simulink model "EV_project"  (R2024a)
settings: Solver=FixedStepAuto  StartTime=0.0  StopTime=250  FixedStep=5e-6  RelTol=1e-6  AbsTol=1e-6
model workspace (MATLAB code in the model file):
  | Rw = 0.2736; % radius of vehicle(m)
  | GVM = 225; % gross vehicle mass(kg)
  | GVW = GVM*9.8; % gross vehicle weight(kg.m/s^2)
  | Crf = 0.012; % coeff of rolling resistance
  | slope_angle = 0; % slope angle in radian
  | Af = 1.73; % frontal Area(m^2)
  | Cd = 0.4; % coeff of drag
  | gear_ratio = 6;
  | trans_eff = 0.95;
  | motor_eff = 0.93;
  | mc_eff = 0.95;
  | Bv = 300; % Battery Voltage(V)
  | Cv = 3.6; % Cell voltage(V)
  | Cc = 31; % Cell capacity(Ah)
  | lap_distance = 0.787; % distance of one lap(km)
  | range = 20; % range of vehicle in single charge
  | time = 60; % time required to complete one lap
  | air_density = 1.225;
libraries: spsDCVoltageSourceLib x1, spsGroundLib x1, slpidlib x1, spsPermanentMagnetSynchronousMachineLib x1, spsThreePhaseVIMeasurementLib x1, spsUniversalBridgeLib x1, simulink x1, spspowerguiLib x1
settings Model: SimulationMode=accelerator  Creator=mohda  LastModifiedBy=MD. ADEEN ASHRAF
settings SolverCC: AlgebraicLoopSolver=TrustRegion
settings RTWCC: GPUComputeCapability=3.5

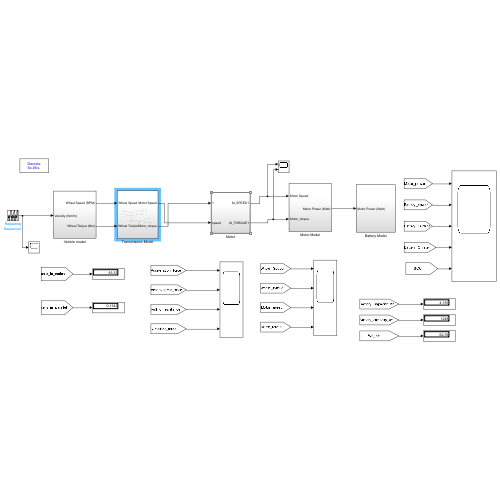
[thumbnail: Simulink's stored preview of the top-level diagram]
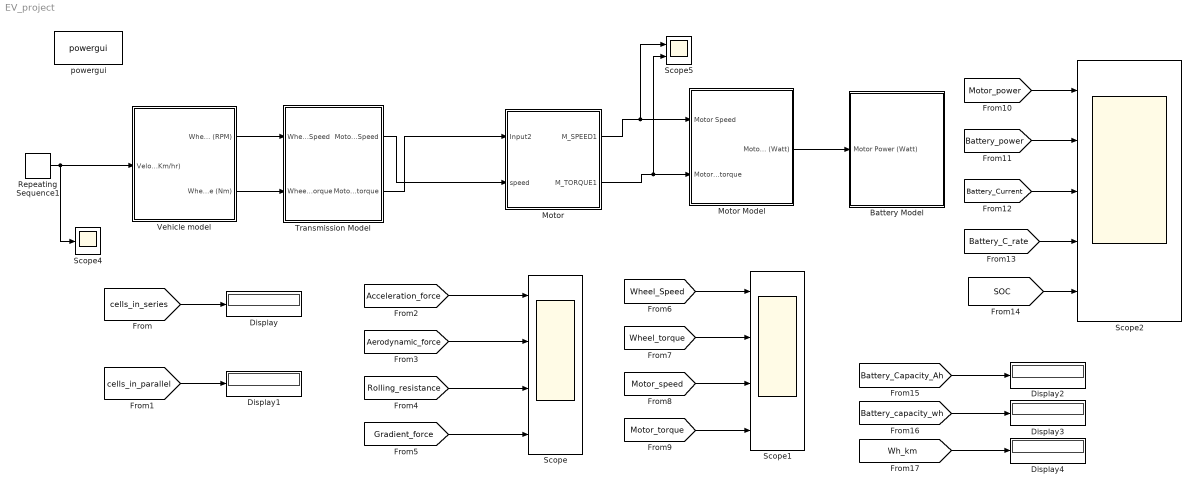
== system EV_project ==
  Battery Model : Subsystem
  Display{,1..4} (5 alike) : Display
  Motor : Subsystem
  Motor Model : Subsystem
  Repeating Sequence1 : simulink/Sources/Repeating Sequence  rep_seq_t=|  rep_seq_y=|
      rep_seq_t=|
      | [0
      | 1
      | 2
      | 3
      | 4
      | 5
      | 6
      | 7
      | 8
      | 9
      | 10
      | 11
      | 12
      | 13
      | 14
      | 15
      | 16
      | 17
      | 18
      | 19
      | 20
      | 21
      | 22
      | 23
      | 24
      | 25
      | 26
      | 27
      | 28
      | 29
      | 30
      | 31
      | 32
      | 33
      | 34
      | 35
      | 36
      | 37
      | 38
      | 39
      | 40
      | 41
      | 42
      | 43
      | 44
      | 45
      | 46
      | 47
      | 48
      | 49
      | 50
      | 51
      | 52
      | 53
      | 54
      | 55
      | 56
      | 57
      | 58
      | 59
      | 60
      | 61
      | 62
      | 63
      | 64
      | 65
      | 66
      | 67
      | 68
      | 69
      | 70
      | 71
      | 72
      | 73
      | 74
      | 75
      | 76
      | 77
      | 78
      | 79
      | 80
      | 81
      | 82
      | 83
      | 84
      | 85
      | 86
      | 87
      | 88
      | 89
      | 90
      | 91
      | 92
      | 93
      | 94
      | 95
      | 96
      | 97
      | 98
      | 99
      | 100
      | 101
      | 102
      | 103
      | 104
      | 105
      | 106
      | 107
      | 108
      | 109
      | 110
      | 111
      | 112
      | 113
      | 114
      | 115
      | 116
      | 117
      | 118
      | 119
      | 120
      | 121
      | 122
      | 123
      | 124
      | 125
      | 126
      | 127
      | 128
      | 129
      | 130
      | 131
      | 132
      | 133
      | 134
      | 135
      | 136
      | 137
      | 138
      | 139
      | 140
      | 141
      | 142
      | 143
      | 144
      | 145
      | 146
      | 147
      | 148
      | 149
      | 150
      | 151
      | 152
      | 153
      | 154
      | 155
      | 156
      | 157
      | 158
      | 159
      | 160
      | 161
      | 162
      | 163
      | 164
      | 165
      | 166
      | 167
      | 168
      | 169
      | 170
      | 171
      | 172
      | 173
      | 174
      | 175
      | 176
      | 177
      | 178
      | 179
      | 180
      | 181
      | 182
      | 183
      | 184
      | 185
      | 186
      | 187
      | 188
      | 189
      | 190
      | 191
      | 192
      | 193
      | 194
      | 195
      | 196
      | 197
      | 198
      | 199
      | 200
      | 201
      | 202
      | 203
      | 204
      | 205
      | 206
      | 207
      | 208
      | 209
      | 210
      | 211
      | 212
      | 213
      | 214
      | 215
      | 216
      | 217
      | 218
      | 219
      | 220
      | 221
      | 222
      | 223
      | 224
      | 225
      | 226
      | 227
      | 228
      | 229
      | 230
      | 231
      | 232
      | 233
      | 234
      | 235
      | 236
      | 237
      | 238
      | 239
      | 240
      | 241
      | 242
      | 243
      | 244
      | 245
      | 246
      | 247
      | 248
      | 249
      | 250 ]
      rep_seq_y=|
      | [0
      | 0
      | 0
      | 0
      | 0
      | 0
      | 0
      | 0
      | 0
      | 0
      | 0
      | 0
      | 3
      | 5.9
      | 8.6
      | 11.5
      | 14.3
      | 16.9
      | 17.3
      | 18.1
      | 20.7
      | 21.7
      | 22.4
      | 22.5
      | 22.1
      | 21.5
      | 20.9
      | 20.4
      | 19.8
      | 17
      | 14.9
      | 14.9
      | 15.2
      | 15.5
      | 16
      | 17.1
      | 19.1
      | 21.1
      | 22.7
      | 22.9
      | 22.7
      | 22.6
      | 21.3
      | 19
      | 17.1
      | 15.8
      | 15.8
      | 17.7
      | 19.8
      | 21.6
      | 23.2
      | 24.2
      | 24.6
      | 24.9
      | 25
      | 25.7
      | 26.1
      | 26.7
      | 27.5
      | 28.6
      | 29.3
      | 29.8
      | 30.1
      | 30.4
      | 30.7
      | 30.7
      | 30.5
      | 30.4
      | 30.3
      | 30.4
      | 30.8
      | 30.4
      | 29.9
      | 29.5
      | 29.8
      | 30.3
      | 30.7
      | 30.9
      | 31
      | 30.9
      | 30.4
      | 29.8
      | 29.9
      | 30.2
      | 30.7
      | 31.2
      | 31.8
      | 32.2
      | 32.4
      | 32.2
      | 31.7
      | 28.6
      | 25.1
      | 21.6
      | 18.1
      | 14.6
      | 11.1
      | 7.6
      | 4.1
      | 0.6
      | 0
      | 0
      | 0
      | 0
      | 0
      | 3.3
      | 6.6
      | 9.9
      | 13.2
      | 16.5
      | 19.8
      | 22.2
      | 24.3
      | 25.8
      | 26.4
      | 25.7
      | 25.1
      | 24.7
      | 25.2
      | 25.4
      | 27.2
      | 26.5
      | 24
      | 22.7
      | 19.4
      | 17.7
      | 17.2
      | 18.1
      | 18.6
      | 20
      | 20.7
      | 21.7
      | 22.4
      | 22.5
      | 22.1
      | 21.5
      | 20.9
      | 20.4
      | 19.8
      | 17
      | 17.1
      | 15.8
      | 15.8
      | 17.7
      | 19.8
      | 21.6
      | 22.2
      | 24.5
      | 24.7
      | 24.8
      | 24.7
      | 24.6
      | 24.6
      | 25.1
      | 25.6
      | 25.7
      | 25.4
      | 24.9
      | 25
      | 25.4
      | 26
      | 26
      | 25.7
      | 26.1
      | 26.7
      | 27.3
      | 30.5
      | 33.5
      | 36.2
      | 37.3
      | 39.3
      | 40.5
      | 42.1
      | 43.5
      | 45.1
      | 46
      | 46.8
      | 47.5
      | 47.5
      | 47.3
      | 47.2
      | 47.2
      | 47.4
      | 47.9
      | 48.5
      | 49.1
      | 49.5
      | 50
      | 50.6
      | 51
      | 51.5
      | 52.2
      | 53.2
      | 54.1
      | 54.6
      | 54.9
      | 55
      | 54.9
      | 54.6
      | 54.6
      | 54.8
      | 55.1
      | 55.5
      | 55.7
      | 56.1
      | 56.3
      | 56.6
      | 56.7
      | 56.7
      | 56.3
      | 56
      | 55
      | 53.4
      | 51.6
      | 51.8
      | 52.1
      | 52.5
      | 53
      | 53.5
      | 54
      | 54.9
      | 55.4
      | 55.6
      | 56
      | 56
      | 55.8
      | 55.2
      | 54.5
      | 53.6
      | 52.5
      | 51.5
      | 50.5
      | 48
      | 44.5
      | 41
      | 37.5
      | 34
      | 30.5
      | 27
      | 23.5
      | 20
      | 16.5
      | 13
      | 9.5
      | 6
      | 2.5
      | 0
      | 0
      | 0
      | 0
      | 0 ]
  Scope : Scope  NumInputPorts=4
  Scope1 : Scope  NumInputPorts=4
  Scope2 : Scope  NumInputPorts=5
  Scope4 : Scope
  Scope5 : Scope  NumInputPorts=2
  Transmission Model : Subsystem
  Vehicle model : Subsystem
  powergui : spspowerguiLib/powergui  Priority=1  SimulationMode=Discrete  SampleTime=5e-6  frequency=60  Iterations=50  frequencyindice=0  Pbase=100e6  ErrMax=1e-4  UnitsV=kV  UnitsW=MW  buscounter=0  FunctionMessages=off  echomessages=off  EnableUseOfTLC=off  CurrentSourceSwitches=off  DisableSnubberDevices=off  DisableRonSwitches=off  DisableVfSwitches=off  DisplayEquations=off  AutomaticDiscreteSolvers=off  SolverType=Tustin/Backward Euler (TBE)  Interpol=off  ExternalGateDelay=off  methode=off  Ts=100  x0status=blocks  SPID=on  SwTol=0  HookPort=off  NonlinearTolerance=1e-4  nMaxIteration=100  ContinueOnMaxIteration=off  RestoreLinks=warning  ResistiveCurrentMeasurement=off  Frange=[0:2:500]  Ylog=off  Xlog=on  ShowGrid=off  save=off  variable=ZData  structure=0  ZoomFFT=off  StartTime=0.0  cycles=1  DisplayStyle=1  fundamental=60  FreqAxis=off  MaxFrequency=1000  frequencyindicesteady=1  RmsSteady=1  display=off
  wires:
  Motor Model/1(Motor Power (Watt)) -> Battery Model/1(Motor Power (Watt))
  [cells_in_series] -> Display/1
  [cells_in_parallel] -> Display1/1
  [Acceleration_force] -> Scope/1
  [Aerodynamic_force] -> Scope/2
  [Rolling_resistance] -> Scope/3
  [Gradient_force] -> Scope/4
  [Wheel_Speed] -> Scope1/1
  [Wheel_torque] -> Scope1/2
  [Motor_speed] -> Scope1/3
  [Motor_torque] -> Scope1/4
  [Battery_C_rate] -> Scope2/4
  [SOC] -> Scope2/5
  [Battery_Current] -> Scope2/3
  [Battery_power] -> Scope2/2
  [Motor_power] -> Scope2/1
  [Battery_Capacity_Ah] -> Display2/1
  [Battery_capacity_wh] -> Display3/1
  [Wh_km] -> Display4/1
  Vehicle model/1(Wheel Speed (RPM)) -> Transmission Model/1(Wheel Speed)
  Vehicle model/2(Wheel Torque (Nm)) -> Transmission Model/2(Wheel Torque)
  Motor/1(M_SPEED1) -> Scope5/1, Motor Model/1(Motor Speed)
  Motor/2(M_TORQUE1) -> Scope5/2, Motor Model/2(Motor_torque)
  Transmission Model/1(Motor Speed) -> Motor/2(speed)
  Transmission Model/2(Motor_torque) -> Motor/1(Input2)
  Repeating Sequence1/1 -> Scope4/1, Vehicle model/1(Velocity (Km/hr))

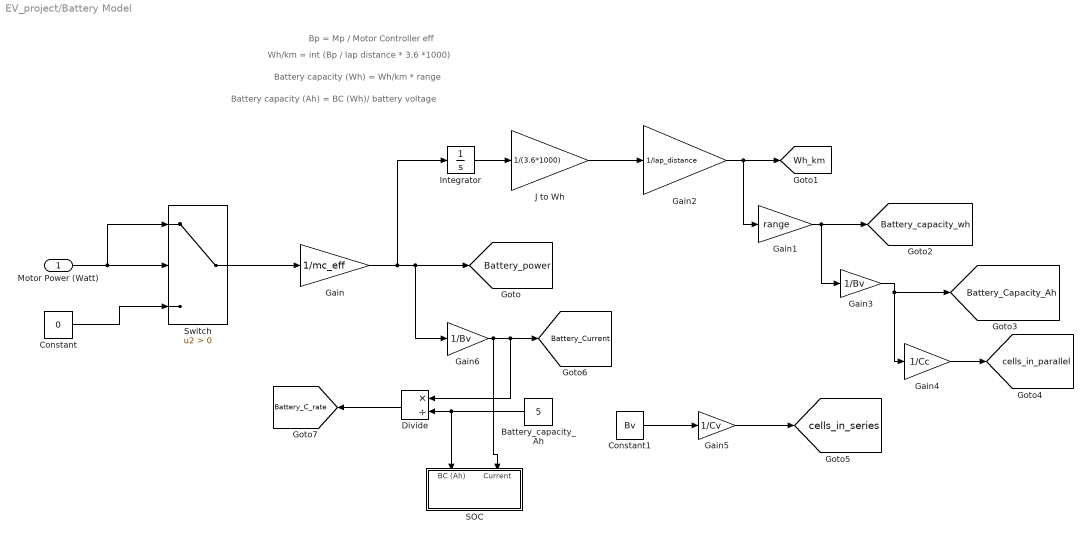
== system EV_project/Battery Model ==
  note: Battery capacity (Ah) = BC (Wh)/ battery voltage
  note: Battery capacity (Wh) = Wh/km * range
  note: Wh/km = int (Bp / lap distance * 3.6 *1000)
  note: Bp = Mp / Motor Controller eff
  Motor Power (Watt) : Inport
  Battery_capacity_Ah : Constant  Value=5
  Constant : Constant  Value=0
  Constant1 : Constant  Value=Bv
  Divide : Product  Inputs=*/
  Gain : Gain  Gain=1/mc_eff
  Gain1 : Gain  Gain=range
  Gain2 : Gain  Gain=1/lap_distance
  Gain3 : Gain  Gain=1/Bv
  Gain4 : Gain  Gain=1/Cc
  Gain5 : Gain  Gain=1/Cv
  Gain6 : Gain  Gain=1/Bv
  Integrator : Integrator
  J to Wh : Gain  Gain=1/(3.6*1000)
  SOC : Subsystem
      settings: PortSchema="{\"entries\":[{\"content\":{\"sides\":[{\"content\":{},\"type\":\"ConnectorPlacement.EquallySpacedRectSide\",\"uuid\":\"2be810da-99f1-4413-b487-e4f7f3ce3b1c\"},{\"content\":{\"side\":\"RIGHT\"},\"type\":\"ConnectorPlacement.EquallySpacedRectSide\",\"uuid\":\"b4550658-4fc6-45c9-b867-461547c61649\"},{\"content\":{\"connectorIds\":[\"In1\",\"In2\"],\"side\":\"TOP\"},\"type\":\"ConnectorPlacement.EquallySpacedRectSide\",\"uuid\":\"a236ffb8-5612-4e8c-b6e9-c7cf7a884809\"}]},\"type\":\"ConnectorPlacement.EquallySpacedConnector\",\"uuid\":\"ea2521ad-76b8-4493-917a-b6fbbcdb85df\"}],\"packageUris\":[\"http://schema.mathworks.com/mf0/Connector/R2020b\"],\"version\":\"1.0\"}"
  Switch : Switch  Criteria=u2 > Threshold  SaturateOnIntegerOverflow=off  InputSameDT=off
  tag scope: Battery_C_rate=global, Battery_Capacity_Ah=global, Battery_Current=global, Battery_capacity_wh=global, Battery_power=global, Wh_km=global, cells_in_parallel=global, cells_in_series=global
  wires:
  Motor Power (Watt)/1 -> Switch/1, Switch/2
  Constant/1 -> Switch/3
  Switch/1 -> Gain/1
  J to Wh/1 -> Gain2/1
  Integrator/1 -> J to Wh/1
  Gain2/1 -> Gain1/1, [Wh_km]
  Gain1/1 -> Gain3/1, [Battery_capacity_wh]
  Gain3/1 -> Gain4/1, [Battery_Capacity_Ah]
  Gain4/1 -> [cells_in_parallel]
  Constant1/1 -> Gain5/1
  Gain5/1 -> [cells_in_series]
  Gain/1 -> Integrator/1, Gain6/1, [Battery_power]
  Gain6/1 -> [Battery_Current], Divide/1, SOC/2(Current)
  Battery_capacity_Ah/1 -> SOC/1(BC (Ah)), Divide/2
  Divide/1 -> [Battery_C_rate]

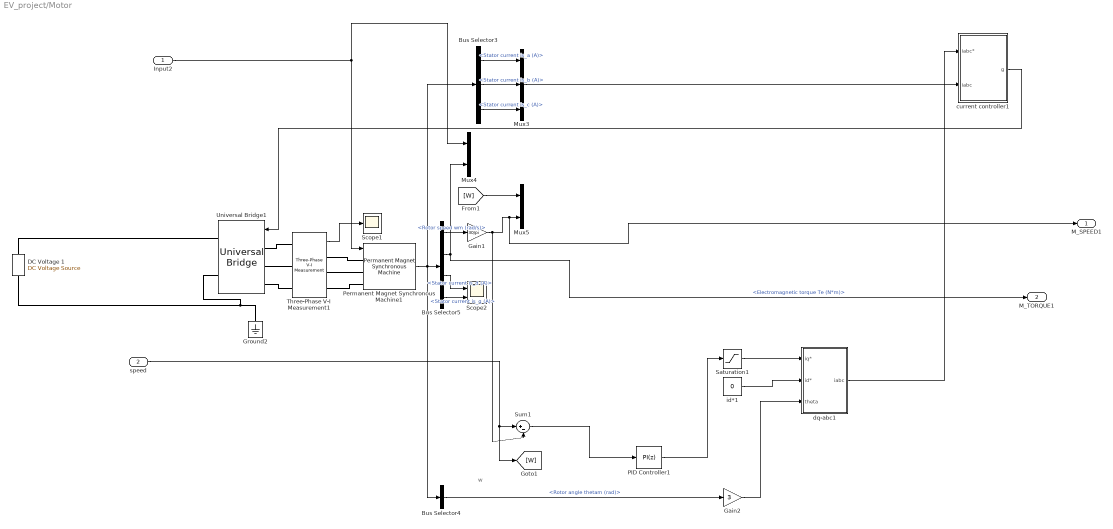
== system EV_project/Motor ==
  note: w
  Input2 : Inport
  speed : Inport  Port=2
  Bus Selector3 : BusSelector  OutputSignals=Stator current is_a (A),Stator current is_b (A),Stator current is_c (A)
  Bus Selector4 : BusSelector  OutputSignals=Rotor angle thetam (rad)
  Bus Selector5 : BusSelector  OutputSignals=Rotor speed wm (rad/s),Electromagnetic torque Te (N*m),Stator current is_d (A),Stator current is_q (A)
  DC Voltage 1 : spsDCVoltageSourceLib/DC Voltage Source  Amplitude=300  Measurements=None
  Gain1 : Gain  Gain=30/pi
  Gain2 : Gain  Gain=3
  Ground2 : spsGroundLib/Ground  LConnTagsString=a
  Mux3 : Mux  Inputs=3
  Mux4 : Mux  Inputs=2
  Mux5 : Mux  Inputs=2
  PID Controller1 : slpidlib/PID Controller  Controller=PI  Form=Ideal  TimeDomain=Discrete-time  UseExternalTs=off  SampleTime=.00001  IntegratorMethod=Forward Euler  FilterMethod=Forward Euler  ControllerParametersSource=internal  P=1  I=.0001  UseKiTs=off  D=0  UseExternalDerivativeSource=off  N=100  UseFilter=on  TunerSelectOption=Transfer Function Based (PID Tuner App)  InitialConditionSource=internal  InitialConditionForIntegrator=0  InitialConditionForFilter=0  DifferentiatorICPrevScaledInput=0  ExternalReset=none  TrackingMode=off  Kt=1  LimitOutput=off  SatLimitsSource=internal  UpperSaturationLimit=inf  LowerSaturationLimit=-inf  LinearizeAsGain=on  AntiWindupMode=none  Kb=1  LimitIntegrator=off  UpperIntegratorSaturationLimit=inf  LowerIntegratorSaturationLimit=-inf  POutMin=[]  POutMax=[]  IOutMin=[]  IOutMax=[]  DOutMin=[]  DOutMax=[]  NOutMin=[]  NOutMax=[]  SumOutMin=[]  SumOutMax=[]  SaturationOutMin=[]  SaturationOutMax=[]  PParamMin=[]  PParamMax=[]  IParamMin=[]  IParamMax=[]  DParamMin=[]  DParamMax=[]  NParamMin=[]  NParamMax=[]  KbParamMin=[]  KbParamMax=[]  KtParamMin=[]  KtParamMax=[]  KbOutMin=[]  KbOutMax=[]  KtOutMin=[]  KtOutMax=[]  IntegratorOutMin=[]  IntegratorOutMax=[]  FilterOutMin=[]  FilterOutMax=[]  SumI1OutMin=[]  SumI1OutMax=[]  SumI2OutMin=[]  SumI2OutMax=[]  SumI3OutMin=[]  SumI3OutMax=[]  SumI4OutMin=[]  SumI4OutMax=[]  SumDOutMin=[]  SumDOutMax=[]  DifferentiatorOutMin=[]  DifferentiatorOutMax=[]  FilterDiffOutCoefMin=[]  FilterDiffOutCoefMax=[]  ReciprocalOutMin=[]  ReciprocalOutMax=[]  SumDenOutMin=[]  SumDenOutMax=[]  SumNumOutMin=[]  SumNumOutMax=[]  DivideOutMin=[]  DivideOutMax=[]  UdiffTsProdOutMin=[]  UdiffTsProdOutMax=[]  NTsProdOutMin=[]  NTsProdOutMax=[]  UintegralTsProdOutMin=[]  UintegralTsProdOutMax=[]  UngainTsProdOutMin=[]  UngainTsProdOutMax=[]  ClampingZeroOutDataTypeStr=Inherit: Inherit via back propagation  ClampingZeroOutMin=[]  ClampingZeroOutMax=[]  FilterDenConstantOutDataTypeStr=Inherit: Inherit via back propagation  FilterDenConstantOutMin=[]  FilterDenConstantOutMax=[]  PCopyOutDataTypeStr=Inherit: Inherit via back propagation  PCopyOutMin=[]  PCopyOutMax=[]  NCopyOutDataTypeStr=Inherit: Inherit via back propagation  NCopyOutMin=[]  NCopyOutMax=[]  IntegratorContinuousStateAttributes=''  IntegratorStateMustResolveToSignalObject=off  IntegratorRTWStateStorageClass=Auto  FilterContinuousStateAttributes=''  FilterStateMustResolveToSignalObject=off  FilterRTWStateStorageClass=Auto  ParallelPVariant=Passthrough  IdealPVariant=InternalParameters  IVariant=InternalParameters  DVariant=Disabled  IntegratorVariant=Discrete  SatVariant=Disabled  AWVariant=Passthrough  PCopyVariant=Disabled  TRVariant=Disabled  FdbkBlocksVariant=Forward  IdealPFdbkVariant=Disabled  SatFdbkVariant=Disabled  DerivativeFilterVariant=Disabled  NVariant=Disabled  NCopyVariant=Disabled_SignalSpec  FilterICVariant=Disabled  IntegratorICVariant=InternalICs  ExternalResetVariant=Disabled  TRSumVariant=Passthrough  SumFdbkVariant=Disabled  SumVariant=Sum_PI  TsampFilterVariant=InternalTs  TsampNgainVariant=Passthrough  TsampIntegralVariant=Disabled_SignalSpec  ExternalSaturationOutDataTypeStr=Inherit: Same as second input  DerivativeSourceVariant=Disabled
  Permanent Magnet Synchronous Machine1 : spsPermanentMagnetSynchronousMachineLib/Permanent Magnet Synchronous Machine  NbPhases=3  FluxDistribution=Sinusoidal  RotorType=Salient-pole  MechanicalLoad=Torque Tm  PresetModel=No  ShowDetailedParameters=on  MeasurementBus=off  Resistance=1.93  Inductance=8.5e-3  dqInductances=[0.0114 ,0.0114]  La=0.000395  MachineConstant=Flux linkage established by magnets (V.s)  Flux=.26603  VoltageCst=144.7575  TorqueCst=1.1971  Flat=120  Mechanical=[0.0011, 0, 3 ,0]  PolePairs=4  InitialConditions=[0,0, 0,0]  InitialConditions5ph=[0 0 0 0 0 0]  RefAngle=90 degrees behind phase A axis (modified Park)  IterativeDiscreteModel=Trapezoidal non iterative  TsBlock=-1  TsPowergui=0
  Saturation1 : Saturate  UpperLimit=12  LowerLimit=-12
  Scope1 : Scope
  Scope2 : Scope  NumInputPorts=2
  Sum1 : Sum  Inputs=|+-
  Three-Phase V-I Measurement1 : spsThreePhaseVIMeasurementLib/Three-Phase V-I Measurement  VoltageMeasurement=phase-to-ground  SetLabelV=off  LabelV=Vabc  Vpu=off  VpuLL=off  CurrentMeasurement=no  SetLabelI=off  LabelI=Iabc  Ipu=on  Pbase=100e6  Vbase=500e3  OutputType=Complex  PhasorSimulation=off  PSBequivalent=0
  Universal Bridge1 : spsUniversalBridgeLib/Universal Bridge  Arms=3  SnubberResistance=1e5  SnubberCapacitance=inf  Device=IGBT / Diodes  Ron=1e-3  Lon=0  ForwardVoltages="[  0  0  ]"  ForwardVoltage=0  GTOparameters=[ 10e-6 , 20e-6 ]  IGBTparameters=[ 1e-6 , 2e-6 ]  Measurements=None  Measurements_2=None  converterType=Rectifier
  current controller1 : Subsystem
  dq-abc1 : Subsystem
  id*1 : Constant  Value=0
  M_SPEED1 : Outport
  M_TORQUE1 : Outport  Port=2
  wires:
  Mux3/1 -> current controller1/2(iabc)
  [W] -> Mux5/1
  Bus Selector3/3 -> Mux3/3  "<Stator current is_c (A)>"
  Permanent Magnet Synchronous Machine1/1 -> Bus Selector4/1, Bus Selector5/1, Bus Selector3/1
  Three-Phase V-I Measurement1/1 -> Scope1/1
  Gain2/1 -> dq-abc1/3(theta)
  Saturation1/1 -> dq-abc1/1(iq*)
  Bus Selector5/1 -> Gain1/1  "<Rotor speed wm (rad/s)>"
  PID Controller1/1 -> Saturation1/1
  Bus Selector4/1 -> Gain2/1  "<Rotor angle thetam (rad)>"
  id*1/1 -> dq-abc1/2(id*)
  Bus Selector3/1 -> Mux3/1  "<Stator current is_a (A)>"
  Gain1/1 -> M_SPEED1/1, Mux5/2, Sum1/2
  Bus Selector5/2 -> Mux4/2, M_TORQUE1/1  "<Electromagnetic torque Te (N*m)>"
  current controller1/1(g) -> Universal Bridge1/1
  speed/1 -> [W], Sum1/1
  dq-abc1/1(iabc) -> current controller1/1(iabc*)
  Sum1/1 -> PID Controller1/1
  Bus Selector3/2 -> Mux3/2  "<Stator current is_b (A)>"
  Input2/1 -> Mux4/1, Permanent Magnet Synchronous Machine1/1
  Bus Selector5/4 -> Scope2/2  "<Stator current is_q (A)>"
  Bus Selector5/3 -> Scope2/1  "<Stator current is_d (A)>"
  connections:
  Universal Bridge1/RConn2 -- DC Voltage 1/LConn1 -- Ground2/LConn1
  Universal Bridge1/RConn1 -- DC Voltage 1/RConn1
  Universal Bridge1/LConn1 -- Three-Phase V-I Measurement1/LConn1
  Universal Bridge1/LConn3 -- Three-Phase V-I Measurement1/LConn3
  Three-Phase V-I Measurement1/RConn1 -- Permanent Magnet Synchronous Machine1/LConn1
  Universal Bridge1/LConn2 -- Three-Phase V-I Measurement1/LConn2
  Three-Phase V-I Measurement1/RConn3 -- Permanent Magnet Synchronous Machine1/LConn3
  Three-Phase V-I Measurement1/RConn2 -- Permanent Magnet Synchronous Machine1/LConn2

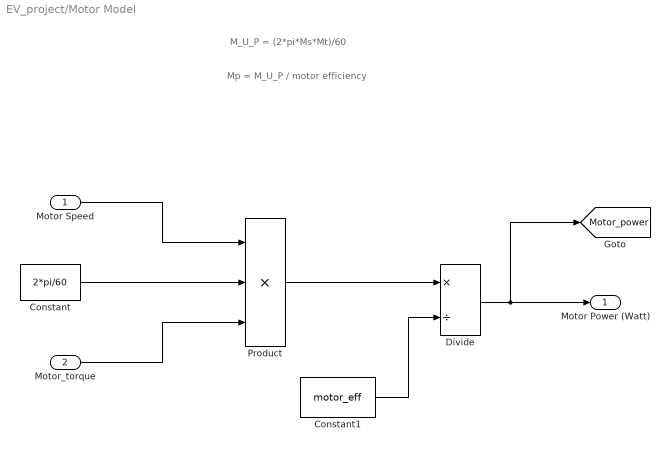
== system EV_project/Motor Model ==
  note: Mp = M_U_P / motor efficiency
  note: M_U_P = (2*pi*Ms*Mt)/60
  Motor Speed : Inport
  Motor_torque : Inport  Port=2
  Constant : Constant  Value=2*pi/60
  Constant1 : Constant  Value=motor_eff
  Divide : Product  Inputs=*/
  Product : Product  Inputs=3
  Motor Power (Watt) : Outport
  tag scope: Motor_power=global
  wires:
  Motor Speed/1 -> Product/1
  Constant/1 -> Product/2
  Motor_torque/1 -> Product/3
  Constant1/1 -> Divide/2
  Product/1 -> Divide/1
  Divide/1 -> [Motor_power], Motor Power (Watt)/1

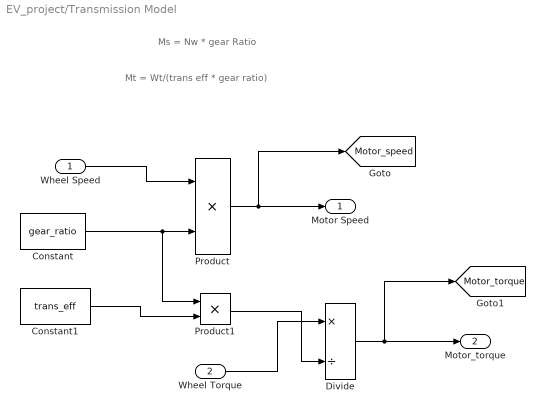
== system EV_project/Transmission Model ==
  note: Mt = Wt/(trans eff * gear ratio)
  note: Ms = Nw * gear Ratio
  Wheel Speed : Inport
  Wheel Torque : Inport  Port=2
  Constant : Constant  Value=gear_ratio
  Constant1 : Constant  Value=trans_eff
  Divide : Product  Inputs=*/
  Product : Product
  Product1 : Product
  Motor Speed : Outport
  Motor_torque : Outport  Port=2
  tag scope: Motor_speed=global, Motor_torque=global
  wires:
  Constant/1 -> Product1/1, Product/2
  Wheel Speed/1 -> Product/1
  Constant1/1 -> Product1/2
  Wheel Torque/1 -> Divide/1
  Product1/1 -> Divide/2
  Product/1 -> [Motor_speed], Motor Speed/1
  Divide/1 -> [Motor_torque], Motor_torque/1

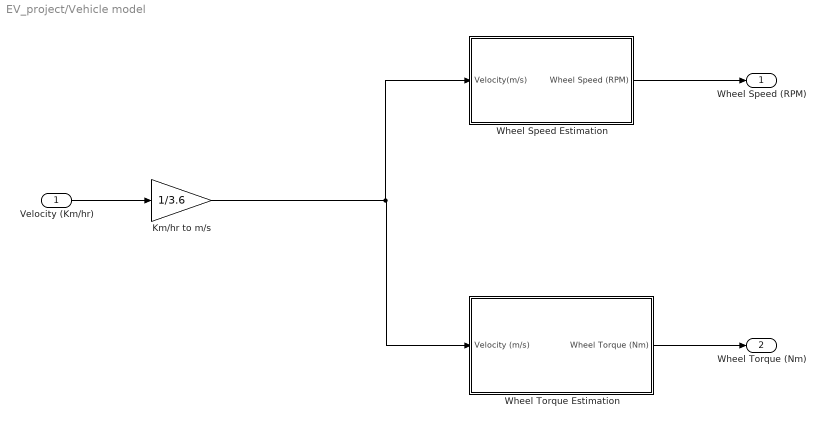
== system EV_project/Vehicle model ==
  Velocity (Km/hr) : Inport
  Km/hr to m/s : Gain  Gain=1/3.6
  Wheel Speed Estimation : Subsystem
  Wheel Torque Estimation : Subsystem
  Wheel Speed (RPM) : Outport
  Wheel Torque (Nm) : Outport  Port=2
  wires:
  Velocity (Km/hr)/1 -> Km/hr to m/s/1
  Wheel Speed Estimation/1(Wheel Speed (RPM)) -> Wheel Speed (RPM)/1
  Wheel Torque Estimation/1(Wheel Torque (Nm)) -> Wheel Torque (Nm)/1
  Km/hr to m/s/1 -> Wheel Speed Estimation/1(Velocity(m/s)), Wheel Torque Estimation/1(Velocity (m/s))

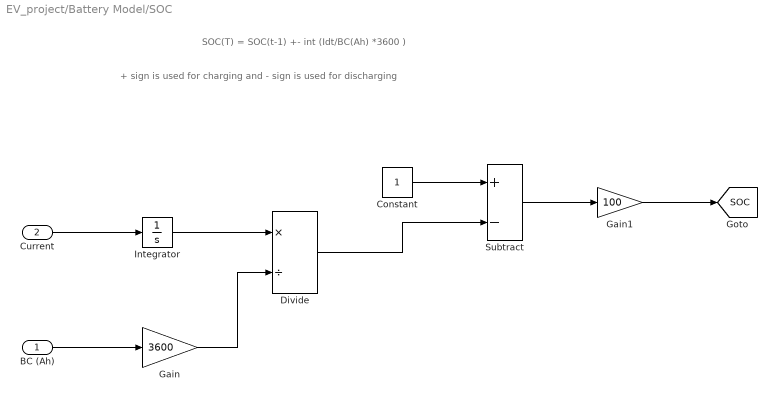
== system EV_project/Battery Model/SOC ==
  note: + sign is used for charging and - sign is used for discharging
  note: SOC(T) = SOC(t-1) +- int (Idt/BC(Ah) *3600 )
  BC (Ah) : Inport
  Current : Inport  Port=2
  Constant : Constant
  Divide : Product  Inputs=*/
  Gain : Gain  Gain=3600
  Gain1 : Gain  Gain=100
  Integrator : Integrator
  Subtract : Sum  Inputs=+-
  tag scope: SOC=global
  wires:
  BC (Ah)/1 -> Gain/1
  Current/1 -> Integrator/1
  Integrator/1 -> Divide/1
  Gain/1 -> Divide/2
  Constant/1 -> Subtract/1
  Divide/1 -> Subtract/2
  Subtract/1 -> Gain1/1
  Gain1/1 -> [SOC]

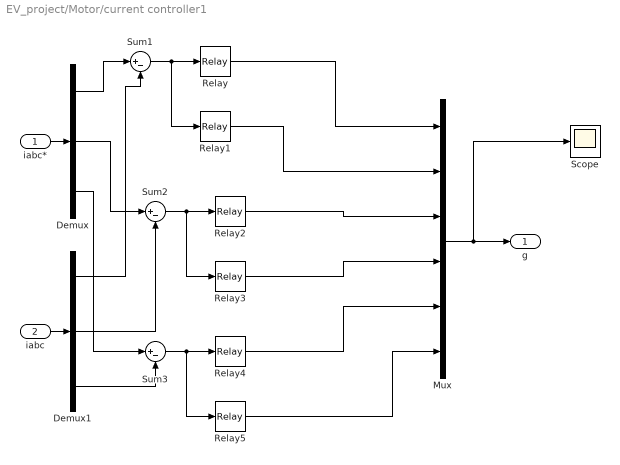
== system EV_project/Motor/current controller1 ==
  iabc* : Inport
  iabc : Inport  Port=2
  Demux : Demux  Outputs=3
  Demux1 : Demux  Outputs=3
  Mux : Mux  Inputs=6
  Relay : Relay  OnSwitchValue=0.1  OffSwitchValue=-0.1
  Relay1 : Relay  OnSwitchValue=0.1  OffSwitchValue=-0.1  OnOutputValue=0  OffOutputValue=1
  Relay2 : Relay  OnSwitchValue=0.1  OffSwitchValue=-0.1
  Relay3 : Relay  OnSwitchValue=0.1  OffSwitchValue=-0.1  OnOutputValue=0  OffOutputValue=1
  Relay4 : Relay  OnSwitchValue=0.1  OffSwitchValue=-0.1
  Relay5 : Relay  OnSwitchValue=0.1  OffSwitchValue=-0.1  OnOutputValue=0  OffOutputValue=1
  Scope : Scope
  Sum1 : Sum  Inputs=|+-
  Sum2 : Sum  Inputs=|+-
  Sum3 : Sum  Inputs=|+-
  g : Outport
  wires:
  Relay3/1 -> Mux/4
  Demux/1 -> Sum1/1
  Relay1/1 -> Mux/2
  Relay5/1 -> Mux/6
  Demux1/3 -> Sum3/2
  Demux1/1 -> Sum1/2
  Demux/3 -> Sum3/1
  Relay2/1 -> Mux/3
  Sum3/1 -> Relay5/1, Relay4/1
  Demux/2 -> Sum2/1
  Demux1/2 -> Sum2/2
  Sum2/1 -> Relay3/1, Relay2/1
  Relay/1 -> Mux/1
  Relay4/1 -> Mux/5
  iabc/1 -> Demux1/1
  iabc*/1 -> Demux/1
  Mux/1 -> Scope/1, g/1
  Sum1/1 -> Relay1/1, Relay/1

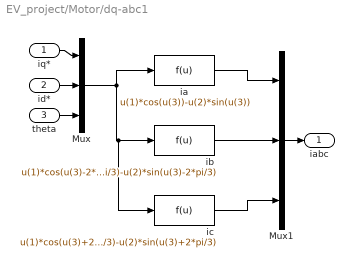
== system EV_project/Motor/dq-abc1 ==
  iq* : Inport
  id* : Inport  Port=2
  theta : Inport  Port=3
  Mux : Mux  Inputs=3
  Mux1 : Mux  Inputs=3
  ia : Fcn  Expr=u(1)*cos(u(3))-u(2)*sin(u(3))
  ib : Fcn  Expr=u(1)*cos(u(3)-2*pi/3)-u(2)*sin(u(3)-2*pi/3)
  ic : Fcn  Expr=u(1)*cos(u(3)+2*pi/3)-u(2)*sin(u(3)+2*pi/3)
  iabc : Outport
  wires:
  ia/1 -> Mux1/1
  ic/1 -> Mux1/3
  ib/1 -> Mux1/2
  id*/1 -> Mux/2
  iq*/1 -> Mux/1
  theta/1 -> Mux/3
  Mux1/1 -> iabc/1
  Mux/1 -> ia/1, ic/1, ib/1

== system EV_project/Vehicle model/Wheel Speed Estimation ==
  note: Nw=(V*60)/(2*pi*Rw)
  Velocity(m/s) : Inport
  Constant : Constant  Value=2*pi*Rw
  Divide : Product  Inputs=*/
  Gain : Gain  Gain=60
  Wheel Speed (RPM) : Outport
  tag scope: Wheel_Speed=global
  wires:
  Velocity(m/s)/1 -> Gain/1
  Gain/1 -> Divide/1
  Constant/1 -> Divide/2
  Divide/1 -> [Wheel_Speed], Wheel Speed (RPM)/1

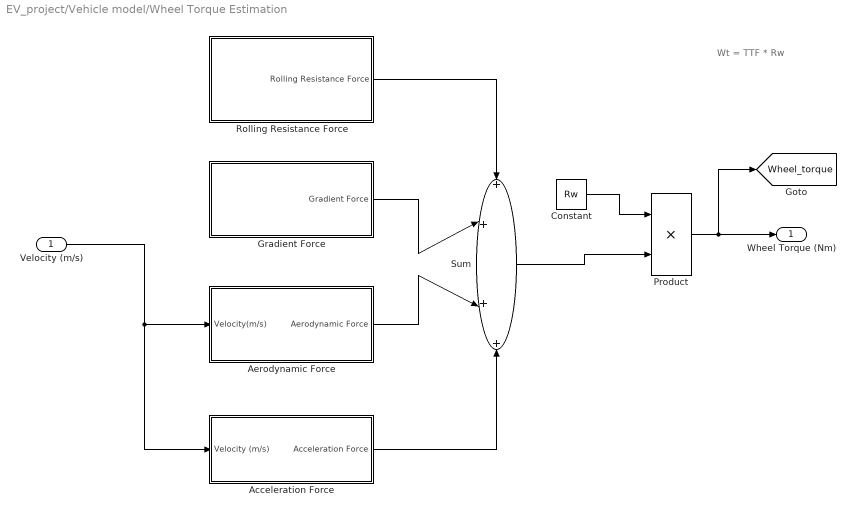
== system EV_project/Vehicle model/Wheel Torque Estimation ==
  note: Wt = TTF * Rw
  Velocity (m/s) : Inport
  Acceleration Force : Subsystem
  Aerodynamic Force : Subsystem
  Constant : Constant  Value=Rw
  Gradient Force : Subsystem
  Product : Product
  Rolling Resistance Force : Subsystem
  Sum : Sum  Inputs=4
  Wheel Torque (Nm) : Outport
  tag scope: Wheel_torque=global
  wires:
  Rolling Resistance Force/1(Rolling Resistance Force) -> Sum/1
  Gradient Force/1(Gradient Force) -> Sum/2
  Aerodynamic Force/1(Aerodynamic Force) -> Sum/3
  Acceleration Force/1(Acceleration Force) -> Sum/4
  Velocity (m/s)/1 -> Acceleration Force/1(Velocity (m/s)), Aerodynamic Force/1(Velocity(m/s))
  Sum/1 -> Product/2
  Constant/1 -> Product/1
  Product/1 -> [Wheel_torque], Wheel Torque (Nm)/1

== system EV_project/Vehicle model/Wheel Torque Estimation/Acceleration Force ==
  note: F acc = GVM * derivative (velocity)
  Velocity (m/s) : Inport
  Constant : Constant  Value=GVM
  Derivative : Derivative
  Product : Product
  Acceleration Force : Outport
  tag scope: Acceleration_force=global
  wires:
  Velocity (m/s)/1 -> Derivative/1
  Derivative/1 -> Product/1
  Constant/1 -> Product/2
  Product/1 -> [Acceleration_force], Acceleration Force/1

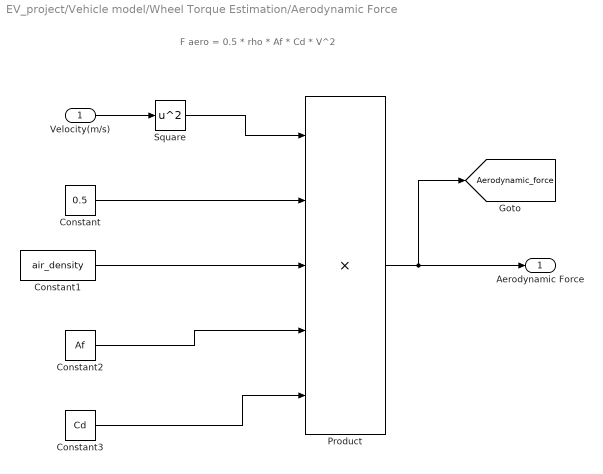
== system EV_project/Vehicle model/Wheel Torque Estimation/Aerodynamic Force ==
  note: F aero = 0.5 * rho * Af * Cd * V^2
  Velocity(m/s) : Inport
  Constant : Constant  Value=0.5
  Constant1 : Constant  Value=air_density
  Constant2 : Constant  Value=Af
  Constant3 : Constant  Value=Cd
  Product : Product  Inputs=5
  Square : Math  Operator=square
  Aerodynamic Force : Outport
  tag scope: Aerodynamic_force=global
  wires:
  Velocity(m/s)/1 -> Square/1
  Square/1 -> Product/1
  Constant/1 -> Product/2
  Constant1/1 -> Product/3
  Constant2/1 -> Product/4
  Constant3/1 -> Product/5
  Product/1 -> [Aerodynamic_force], Aerodynamic Force/1

== system EV_project/Vehicle model/Wheel Torque Estimation/Gradient Force ==
  note: theta is in radian
  note: F grad = GVW * sin (theta)
  Constant : Constant  Value=GVW
  Constant1 : Constant  Value=slope_angle
  Product : Product
  Sin : Trigonometry
  Gradient Force : Outport
  tag scope: Gradient_force=global
  wires:
  Constant1/1 -> Sin/1
  Constant/1 -> Product/1
  Sin/1 -> Product/2
  Product/1 -> [Gradient_force], Gradient Force/1

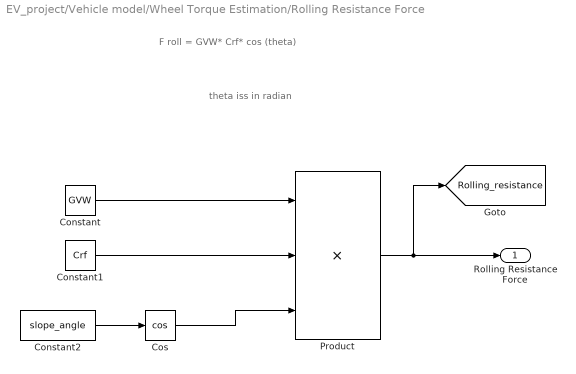
== system EV_project/Vehicle model/Wheel Torque Estimation/Rolling Resistance Force ==
  note: theta iss in radian
  note: F roll = GVW* Crf* cos (theta)
  Constant : Constant  Value=GVW
  Constant1 : Constant  Value=Crf
  Constant2 : Constant  Value=slope_angle
  Cos : Trigonometry  Operator=cos
  Product : Product  Inputs=3
  Rolling Resistance Force : Outport
  tag scope: Rolling_resistance=global
  wires:
  Constant2/1 -> Cos/1
  Constant/1 -> Product/1
  Constant1/1 -> Product/2
  Cos/1 -> Product/3
  Product/1 -> [Rolling_resistance], Rolling Resistance Force/1
